simulink model "OFDM_Tx_Rx_Loopback"  (R2020a)
settings: Solver=FixedStepDiscrete  StartTime=0.0  StopTime=inf  RelTol=1e-3
InitFcn:
  | % Set parameters
  | fs = 200e3;
  | 
  | % Load all required variables
  | load('read_addr_data');
  | load('read_addr_cp');
  | load('read_addr_pream');
  | load('read_addr_rx');
  | load('pilot');
  | load('LTSfreq');
  | load('STSfreq');
  | load('LTSread');
  | load('STSread');
  | load('bpsk');
  | load('qpsk');
  | load('qam16');
values from neighbouring files (symbols this model uses):
  bpsk = [0 0 1 1 1 1 0 0 1 0 1 0 ... (48 elements, 48x1)]    [bpsk.mat]
  qam16 = [12 5 10 3 14 8 1 10 8 7 2 13 ... (48 elements, 48x1)]    [qam16.mat]
  qpsk = [1 2 1 2 2 2 3 1 1 3 1 0 ... (48 elements, 48x1)]    [qpsk.mat]
  STSfreq = [0 0 0 0 0 0 0 0 1 0 0 0 ... (64 elements, 1x64)]    [STSfreq.mat]
undefined symbols (not defined in the file or in its folder): data3, LTSfreq, LTSread, pilot, read_addr_cp, read_addr_data, read_addr_pream, read_addr_rx, STSread
libraries: hdlsllib x54, simulink x27, dsphdlxfrm x2, dsphdlsigops x1, dsphdlmathfun x1
(part 1 of 4)
settings Model: Creator=njb13206  LastModifiedBy=njb13206
settings OptimizationCC: BlockReduction=off  ConditionallyExecuteInputs=off  DefaultParameterBehavior=Inlined
settings DebuggingCC: AlgebraicLoopMsg=error  IntegerOverflowMsg=none  ParameterPrecisionLossMsg=none  IntegerSaturationMsg=none
settings HardwareCC: ProdBitPerPointer=32  ProdBitPerSizeT=32  ProdBitPerPtrDiffT=32  ProdLargestAtomicFloat=None  ProdIntDivRoundTo=Undefined  ProdEndianess=Unspecified  ProdWordSize=32  ProdHWDeviceType=ASIC/FPGA->ASIC/FPGA  TargetBitPerPointer=64  TargetBitPerSizeT=64  TargetBitPerPtrDiffT=64  TargetLongLongMode=on  TargetIntDivRoundTo=Zero  TargetEndianess=LittleEndian  TargetWordSize=64  TargetHWDeviceType=Custom Processor->MATLAB Host Computer  ProdEqTarget=off

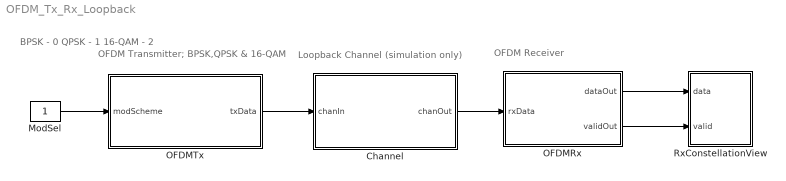
== system OFDM_Tx_Rx_Loopback ==
  note: OFDM Receiver
  note: Loopback Channel (simulation only)
  note: OFDM Transmitter; BPSK,QPSK & 16-QAM
  note: BPSK - 0
      | QPSK - 1
      | 16-QAM - 2
  "Channel " : Subsystem
  ModSel : Constant  OutDataTypeStr=fixdt(0,2,0)  SampleTime=1/fs
  OFDMRx : Subsystem
  OFDMTx : Subsystem
  RxConstellationView : Subsystem
  wires:
  "Channel "/1(chanOut) -> OFDMRx/1(rxData)
  OFDMTx/1(txData) -> "Channel "/1(chanIn)
  OFDMRx/1(dataOut) -> RxConstellationView/1(data)
  OFDMRx/2(validOut) -> RxConstellationView/2(valid)
  ModSel/1 -> OFDMTx/1(modScheme)

== system OFDM_Tx_Rx_Loopback/Channel  ==
  chanIn : Inport
  Delay : Delay  DelayLength=5
  Gain : Gain  Gain=0.1  OutDataTypeStr=fixdt(1,16,14)
  chanOut : Outport  VectorParamsAs1DForOutWhenUnconnected=off
  wires:
  Delay/1 -> chanOut/1
  chanIn/1 -> Gain/1
  Gain/1 -> Delay/1

== system OFDM_Tx_Rx_Loopback/OFDMRx ==
  note: One Tap Equaliser
  note: FFT Demodulation
  note: Timing and Frequency
      | synchronisation
  rxData : Inport
  ChannelEstEq : Subsystem
  FFT : Subsystem
  Synchronisation : Subsystem
  dataOut : Outport  VectorParamsAs1DForOutWhenUnconnected=off
  validOut : Outport  Port=2  VectorParamsAs1DForOutWhenUnconnected=off
  wires:
  rxData/1 -> Synchronisation/1(dataIn)
  FFT/1(dataOut) -> ChannelEstEq/1(dataIn)
  FFT/3(preambleValidOut) -> ChannelEstEq/3(preambleValid)
  FFT/2(dataValidOut) -> ChannelEstEq/2(dataValid)
  Synchronisation/1(DataOut) -> FFT/1(dataIn)
  Synchronisation/2(FFTValidOut) -> FFT/2(FFTValidIn)
  Synchronisation/3(dataValid) -> FFT/3(dataValid)
  Synchronisation/4(preambleValid) -> FFT/4(preambleValid)
  ChannelEstEq/1(dataOut) -> dataOut/1
  ChannelEstEq/2(dataValidOut) -> validOut/1

== system OFDM_Tx_Rx_Loopback/OFDMTx ==
  note: Generate random integers, M-QAM symbol mapping and sub-carrier
      | mapping.
  note: Add Cyclic Prefix
  note: Create OFDM symbols using
      | IFFT
  modScheme : Inport
  CPAdd : Subsystem
  Constant : Constant  OutDataTypeStr=boolean  SampleTime=1/fs
  ControlSignalGenerator : Subsystem
  DataGenerator : Subsystem
  IFFT : Subsystem
  SCMapper : Subsystem
  txData : Outport  VectorParamsAs1DForOutWhenUnconnected=off
  wires:
  DataGenerator/1(dataOut) -> SCMapper/1(dataIn)
  DataGenerator/2(preambValOut) -> SCMapper/2(preambValid)
  DataGenerator/3(dataValidOut) -> SCMapper/3(dataValid)
  SCMapper/1(dataOut) -> IFFT/1(dataIn)
  SCMapper/2(preambValidOut) -> IFFT/2(preambleValidIn)
  SCMapper/3(dataValidOut) -> IFFT/3("dataValidIn ")
  IFFT/1(dataOut) -> CPAdd/1(dataIn)
  IFFT/2(preambValidOut) -> CPAdd/2(preambValid)
  IFFT/3(dataValidOut) -> CPAdd/3(dataValid)
  CPAdd/1(dataOut) -> txData/1
  ControlSignalGenerator/1(dataValid) -> DataGenerator/2(dataValid)
  ControlSignalGenerator/2(preambleValid) -> DataGenerator/3(preambleValid)
  ControlSignalGenerator/3(dataReady) -> DataGenerator/4(dataReady)
  ControlSignalGenerator/4(PilotValid) -> DataGenerator/5(pilotValid)
  modScheme/1 -> DataGenerator/1(modScheme)
  Constant/1 -> ControlSignalGenerator/1(enable)

== system OFDM_Tx_Rx_Loopback/RxConstellationView ==
  data : Inport
  valid : Inport  Port=2
  Constant : Constant  Value=NaN + 1i*NaN  OutDataTypeStr=double  SampleTime=-1
  Constellation Diagram : ConstellationDiagram
  Switch : Switch  Criteria=u2 ~= 0
  wires:
  Switch/1 -> Constellation Diagram/1
  Constant/1 -> Switch/3
  valid/1 -> Switch/2
  data/1 -> Switch/1

== system OFDM_Tx_Rx_Loopback/OFDMRx/ChannelEstEq ==
  dataIn : Inport
  dataValid : Inport  Port=2
  preambleValid : Inport  Port=3
  ChannelEstimate : Subsystem
  DataArrange : Subsystem
  Delay : Delay  DelayLength=6
  Equalise : Subsystem
  dataOut : Outport  VectorParamsAs1DForOutWhenUnconnected=off
  dataValidOut : Outport  Port=2  VectorParamsAs1DForOutWhenUnconnected=off
  wires:
  ChannelEstimate/2(dataValidOut) -> Equalise/3(dataValidIn)
  ChannelEstimate/1(chEstOut) -> Equalise/2(chEstIn)
  Delay/1 -> Equalise/1(dataInEq)
  dataIn/1 -> ChannelEstimate/1(dataIn), Delay/1
  preambleValid/1 -> ChannelEstimate/2(preambleValid)
  dataValid/1 -> ChannelEstimate/3(dataValidIn)
  Equalise/1(dataOutEq) -> DataArrange/1(dataIn)
  Equalise/2(dataValidOut) -> DataArrange/2(validIn)
  DataArrange/1(dataOut) -> dataOut/1
  DataArrange/2(validOut) -> dataValidOut/1

== system OFDM_Tx_Rx_Loopback/OFDMRx/FFT ==
  dataIn : Inport
  FFTValidIn : Inport  Port=2
  dataValid : Inport  Port=3
  preambleValid : Inport  Port=4
  Delay1 : Delay  DelayLength=173
  Delay2 : Delay  DelayLength=173
  FFT HDL Optimized : dsphdlxfrm/FFT HDL Optimized  FFTLength=64  Architecture=Streaming Radix 2^2  ComplexMultiplication=Use 4 multipliers and 2 adders  BitReversedOutput=off  BitReversedInput=off  Normalize=off  SimulateUsing=Code generation  RoundingMethod=Floor  ResetInputPort=off  StartOutputPort=off  EndOutputPort=off
      settings: SourceProductBaseCode=DS
  Terminator : Terminator
  dataOut : Outport  VectorParamsAs1DForOutWhenUnconnected=off
  dataValidOut : Outport  Port=2  VectorParamsAs1DForOutWhenUnconnected=off
  preambleValidOut : Outport  Port=3  VectorParamsAs1DForOutWhenUnconnected=off
  wires:
  FFTValidIn/1 -> FFT HDL Optimized/2
  dataIn/1 -> FFT HDL Optimized/1
  Delay2/1 -> dataValidOut/1
  Delay1/1 -> preambleValidOut/1
  FFT HDL Optimized/1 -> dataOut/1
  FFT HDL Optimized/2 -> Terminator/1
  dataValid/1 -> Delay2/1
  preambleValid/1 -> Delay1/1

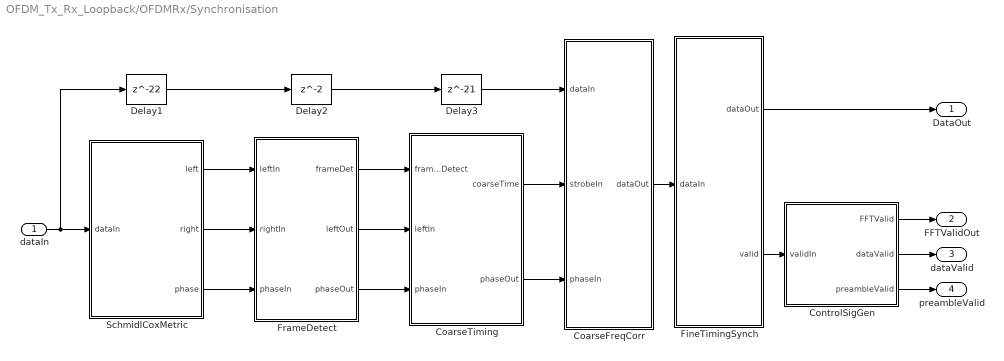
== system OFDM_Tx_Rx_Loopback/OFDMRx/Synchronisation ==
  dataIn : Inport
  CoarseFreqCorr : Subsystem
  CoarseTiming : Subsystem
  ControlSigGen : Subsystem
  Delay1 : Delay  DelayLength=22  InputProcessing=Columns as channels (frame based)
  Delay2 : Delay  InputProcessing=Columns as channels (frame based)
  Delay3 : Delay  DelayLength=21  InputProcessing=Columns as channels (frame based)
  FineTimingSynch : Subsystem
  FrameDetect : Subsystem
  "SchmidlCoxMetric " : Subsystem
  DataOut : Outport  VectorParamsAs1DForOutWhenUnconnected=off
  FFTValidOut : Outport  Port=2  VectorParamsAs1DForOutWhenUnconnected=off
  dataValid : Outport  Port=3  VectorParamsAs1DForOutWhenUnconnected=off
  preambleValid : Outport  Port=4  VectorParamsAs1DForOutWhenUnconnected=off
  wires:
  Delay1/1 -> Delay2/1
  "SchmidlCoxMetric "/3(phase) -> FrameDetect/3(phaseIn)
  "SchmidlCoxMetric "/2(right) -> FrameDetect/2(rightIn)
  FineTimingSynch/1(dataOut) -> DataOut/1
  FrameDetect/2(leftOut) -> CoarseTiming/2(leftIn)
  Delay2/1 -> Delay3/1
  FrameDetect/1(frameDet) -> CoarseTiming/1(frameDetect)
  FrameDetect/3(phaseOut) -> CoarseTiming/3(phaseIn)
  CoarseTiming/1(coarseTime) -> CoarseFreqCorr/2(strobeIn)
  dataIn/1 -> "SchmidlCoxMetric "/1(dataIn), Delay1/1
  Delay3/1 -> CoarseFreqCorr/1(dataIn)
  "SchmidlCoxMetric "/1(left) -> FrameDetect/1(leftIn)
  CoarseFreqCorr/1(dataOut) -> FineTimingSynch/1(dataIn)
  CoarseTiming/2(phaseOut) -> CoarseFreqCorr/3(phaseIn)
  ControlSigGen/1(FFTValid) -> FFTValidOut/1
  FineTimingSynch/2(valid) -> ControlSigGen/1(validIn)
  ControlSigGen/2(dataValid) -> dataValid/1
  ControlSigGen/3(preambleValid) -> preambleValid/1

== system OFDM_Tx_Rx_Loopback/OFDMTx/CPAdd ==
  dataIn : Inport
  preambValid : Inport  Port=2
  dataValid : Inport  Port=3
  DataExtend : Subsystem
  LTFExtend : Subsystem
  Mux2 : MATLAB Function  TreatAsAtomicUnit=on
  STFExtend : Subsystem
  dataOut : Outport  VectorParamsAs1DForOutWhenUnconnected=off
  wires:
  preambValid/1 -> LTFExtend/2(preambVal), STFExtend/2(preambVal)
  dataIn/1 -> DataExtend/1(dataIn), LTFExtend/1(data), STFExtend/1(data)
  STFExtend/1(STFExtendOut) -> Mux2/1(sts)
  STFExtend/2(STFValidOut) -> Mux2/2(stsval)
  LTFExtend/1(LTFExtendOut) -> Mux2/3(lts)
  LTFExtend/2(LTFValidOut) -> Mux2/4(ltsval)
  DataExtend/1(dataOut) -> Mux2/5(data)
  DataExtend/2(dataValidOut) -> Mux2/6(dataval)
  Mux2/1(dataOut) -> dataOut/1
  dataValid/1 -> DataExtend/2(dataValid)

== system OFDM_Tx_Rx_Loopback/OFDMTx/ControlSignalGenerator ==
  enable : Inport
  PreamValidGen : Subsystem
  dataReadyGen : Subsystem
  dataValidGen : Subsystem
  pilotValidGen : Subsystem
  dataValid : Outport
  preambleValid : Outport  Port=2
  dataReady : Outport  Port=3
  PilotValid : Outport  Port=4
  wires:
  enable/1 -> dataValidGen/2(enable), PreamValidGen/1(enable)
  dataReadyGen/1(y) -> dataReady/1
  pilotValidGen/1(y) -> PilotValid/1
  PreamValidGen/1(y) -> preambleValid/1, dataValidGen/1(y)
  dataValidGen/1(valOut) -> pilotValidGen/1(enb), dataReadyGen/1(enb), dataValid/1

== system OFDM_Tx_Rx_Loopback/OFDMTx/DataGenerator ==
  modScheme : Inport
  dataValid : Inport  Port=2
  preambleValid : Inport  Port=3
  dataReady : Inport  Port=4
  pilotValid : Inport  Port=5
  Data Multiplexer : MATLAB Function  TreatAsAtomicUnit=on
  LTSfreq : Subsystem
  PilotGen : Subsystem
  STSFreq : Subsystem
  SymbolsGen : Subsystem
  dataOut : Outport  VectorParamsAs1DForOutWhenUnconnected=off
  preambValOut : Outport  Port=2  VectorParamsAs1DForOutWhenUnconnected=off
  dataValidOut : Outport  Port=3  VectorParamsAs1DForOutWhenUnconnected=off
  wires:
  SymbolsGen/1(symbsOut) -> Data Multiplexer/1(symbols)
  LTSfreq/1(ltsFreq) -> Data Multiplexer/7(lts)
  LTSfreq/2(ltsVal) -> Data Multiplexer/8(ltsval)
  PilotGen/1(pilotOut) -> Data Multiplexer/3(pilots)
  STSFreq/1(stsFreq) -> Data Multiplexer/5(sts)
  STSFreq/2(stsVal) -> Data Multiplexer/6(stsval)
  Data Multiplexer/1(data) -> dataOut/1
  dataValid/1 -> dataValidOut/1, PilotGen/1(dataValidIn)
  preambleValid/1 -> STSFreq/1(preamVal), LTSfreq/1(preambVal), preambValOut/1
  dataReady/1 -> SymbolsGen/2(valid), Data Multiplexer/2(dataready)
  pilotValid/1 -> PilotGen/2(pilotValidIn), Data Multiplexer/4(pval)
  modScheme/1 -> SymbolsGen/1(modScheme)

== system OFDM_Tx_Rx_Loopback/OFDMTx/IFFT ==
  dataIn : Inport
  preambleValidIn : Inport  Port=2
  "dataValidIn " : Inport  Port=3
  Delay : Delay  DelayLength=173  InitialCondition=0  UseCircularBuffer=on
  Delay1 : Delay  DelayLength=173  InitialCondition=0  UseCircularBuffer=on
  IFFT HDL Optimized : dsphdlxfrm/IFFT HDL Optimized  FFTLength=64  Architecture=Streaming Radix 2^2  ComplexMultiplication=Use 3 multipliers and 5 adders  BitReversedOutput=off  BitReversedInput=off  Normalize=on  SimulateUsing=Code generation  RoundingMethod=Floor  ResetInputPort=off  StartOutputPort=off  EndOutputPort=off
      settings: SourceProductBaseCode=DS
  IFFTValid : Subsystem
  Terminator : Terminator
  dataOut : Outport  VectorParamsAs1DForOutWhenUnconnected=off
  preambValidOut : Outport  Port=2  VectorParamsAs1DForOutWhenUnconnected=off
  dataValidOut : Outport  Port=3  VectorParamsAs1DForOutWhenUnconnected=off
  wires:
  dataIn/1 -> IFFT HDL Optimized/1
  IFFT HDL Optimized/2 -> Terminator/1
  "dataValidIn "/1 -> IFFTValid/2(dataValid), Delay1/1
  IFFTValid/1(ifftValid) -> IFFT HDL Optimized/2
  preambleValidIn/1 -> IFFTValid/1(preambleValid), Delay/1
  Delay/1 -> preambValidOut/1
  Delay1/1 -> dataValidOut/1
  IFFT HDL Optimized/1 -> dataOut/1

== system OFDM_Tx_Rx_Loopback/OFDMTx/SCMapper ==
  dataIn : Inport
  preambValid : Inport  Port=2
  dataValid : Inport  Port=3
  DataMapper : Subsystem
  Mux2 : MATLAB Function  TreatAsAtomicUnit=on
  PremableMapper : Subsystem
  dataOut : Outport  VectorParamsAs1DForOutWhenUnconnected=off
  preambValidOut : Outport  Port=2  VectorParamsAs1DForOutWhenUnconnected=off
  dataValidOut : Outport  Port=3  VectorParamsAs1DForOutWhenUnconnected=off
  wires:
  PremableMapper/1(preambleShiftOut) -> Mux2/1(preamb)
  PremableMapper/2(preambValOut) -> preambValidOut/1, Mux2/2(preambVal)
  DataMapper/1(dataOut) -> Mux2/3(data)
  DataMapper/2(dataValidOut) -> dataValidOut/1, Mux2/4(dataVal)
  dataIn/1 -> DataMapper/1(dataIn), PremableMapper/1(data)
  preambValid/1 -> PremableMapper/2(preambVal)
  dataValid/1 -> DataMapper/2(dataValid)
  Mux2/1(dataOut) -> dataOut/1

== system OFDM_Tx_Rx_Loopback/OFDMRx/ChannelEstEq/ChannelEstimate ==
  note: Note the preamble symbols do not pass this point.
  note: Write averaged channel estimate to RAM and read out when data is valid
      | for equalisation of successive OFDM symbols.
  note: Get and store the channel estimate using the two
      | repetitions of the L-LTF
  dataIn : Inport
  preambleValid : Inport  Port=2
  dataValidIn : Inport  Port=3
  ChanEst : Subsystem
  Delay : Delay  DelayLength=5
  Delay1 : Delay  DelayLength=5
  Delay2 : Delay  DelayLength=1
  Dual Port RAM1 : hdlsllib/HDL RAMs/Dual Port RAM  ram_size=6
      settings: SourceProductBaseCode=SL
  HDL Counter3 : hdlsllib/Sources/HDL Counter  CountType=Count limited  CountInit=0  CountStep=1  CountMax=63  CountFromType=Initial value  CountFrom=0  CountResetPort=off  CountLoadPort=off  CountEnbPort=on  CountDirPort=off  CountDataType=Unsigned  CountWordLen=6  CountFracLen=0  CountSampTime=1
  Terminator : Terminator
  WriteEnbAddrGen : Subsystem
  chEstOut : Outport  VectorParamsAs1DForOutWhenUnconnected=off
  dataValidOut : Outport  Port=2  VectorParamsAs1DForOutWhenUnconnected=off
  wires:
  HDL Counter3/1 -> Dual Port RAM1/4
  Dual Port RAM1/2 -> chEstOut/1
  Delay2/1 -> dataValidOut/1
  preambleValid/1 -> ChanEst/2(PreambValidIn), Delay/1
  dataIn/1 -> ChanEst/1(ChanEstIn)
  ChanEst/1(ChEstOut) -> Dual Port RAM1/1
  dataValidIn/1 -> Delay1/1
  Delay1/1 -> HDL Counter3/1, Delay2/1
  Delay/1 -> WriteEnbAddrGen/1(In1)
  WriteEnbAddrGen/1(Out1) -> Dual Port RAM1/2
  WriteEnbAddrGen/2(Out2) -> Dual Port RAM1/3
  Dual Port RAM1/1 -> Terminator/1

== system OFDM_Tx_Rx_Loopback/OFDMRx/ChannelEstEq/DataArrange ==
  dataIn : Inport
  validIn : Inport  Port=2
  Compare To Constant4 : simulink/Logic and Bit Operations/Compare To Constant  relop=>=  const=17  OutDataTypeStr=boolean
  Compare To Constant5 : simulink/Logic and Bit Operations/Compare To Constant  relop=<=  const=64  OutDataTypeStr=boolean
  Data Type Conversion : DataTypeConversion  OutDataTypeStr=fixdt(1,16,14)
  Logical Operator2 : Logic  IconShape=distinctive  AllPortsSameDT=off  OutDataTypeStr=boolean
  SCReArrange : Subsystem
  SampleCounter : Subsystem
  dataOut : Outport
  validOut : Outport  Port=2
  wires:
  SampleCounter/1(Sample_Cnt) -> Compare To Constant4/1, Compare To Constant5/1
  Compare To Constant4/1 -> Logical Operator2/1
  Compare To Constant5/1 -> Logical Operator2/2
  SCReArrange/2(DataValidOut) -> SampleCounter/1(Valid_In)
  dataIn/1 -> SCReArrange/1(DataIn)
  validIn/1 -> SCReArrange/2(DataValidIn)
  SCReArrange/1(DataOut) -> Data Type Conversion/1
  Logical Operator2/1 -> validOut/1
  Data Type Conversion/1 -> dataOut/1

== system OFDM_Tx_Rx_Loopback/OFDMRx/ChannelEstEq/Equalise ==
  dataInEq : Inport
  chEstIn : Inport  Port=2
  dataValidIn : Inport  Port=3
  Abs2 : Subsystem
  Complex Mult : Subsystem
  Delay1 : Delay
  Delay8 : Delay  DelayLength=3
  Divide : Subsystem
  dataOutEq : Outport  VectorParamsAs1DForOutWhenUnconnected=off
  dataValidOut : Outport  Port=2  VectorParamsAs1DForOutWhenUnconnected=off
  wires:
  dataValidIn/1 -> Delay8/1
  chEstIn/1 -> Abs2/1(ChEstIn), Complex Mult/2(In2)
  dataInEq/1 -> Complex Mult/1(In1)
  Complex Mult/1(Out1) -> Divide/1(In1)
  Abs2/1(Out1) -> Divide/2(In2)
  Divide/1(Out1) -> dataOutEq/1
  Delay8/1 -> Delay1/1
  Delay1/1 -> dataValidOut/1

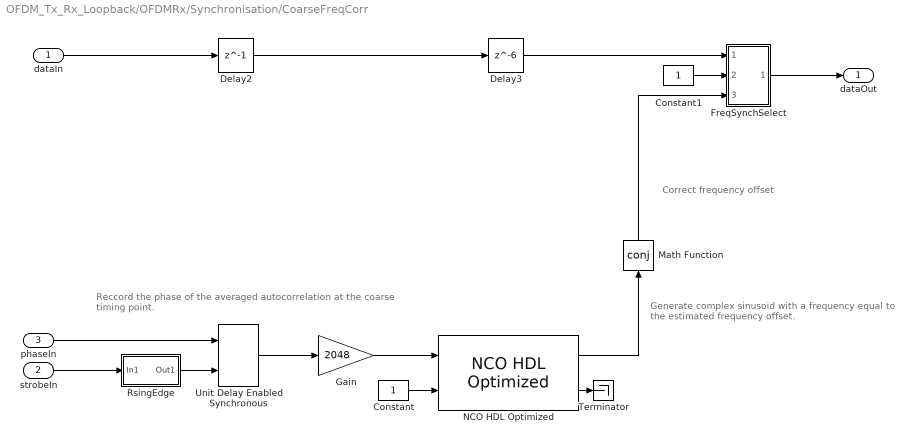
== system OFDM_Tx_Rx_Loopback/OFDMRx/Synchronisation/CoarseFreqCorr ==
  note: Generate complex sinusoid with a frequency equal
      | to the estimated frequency offset.
  note: Correct frequency offset
  note: Reccord the phase of the averaged autocorrelation at the coarse
      | timing point.
  dataIn : Inport
  strobeIn : Inport  Port=2
  phaseIn : Inport  Port=3
  Constant : Constant  VectorParams1D=off  OutDataTypeStr=boolean  SampleTime=1/fs
  Constant1 : Constant  OutDataTypeStr=fixdt(0,1,0)  SampleTime=1/fs
  Delay2 : Delay  DelayLength=1
  Delay3 : Delay  DelayLength=6
  FreqSynchSelect : Subsystem
  Gain : Gain  Gain=2048  OutDataTypeStr=uint16
  Math Function : Math  Operator=conj  SignedPower=on  RndMeth=Zero  SaturateOnIntegerOverflow=on
  NCO HDL Optimized : dsphdlsigops/NCO HDL Optimized  PhaseIncrementSource=Input port  PhaseIncrement=100  PhaseOffsetSource=Property  PhaseOffset=0  DitherSource=Property  NumDitherBits=4  SamplesPerFrame=1  LUTCompress=on  ResetAction=off  Waveform=Complex exponential  PhasePort=off  SimulateUsing=Code generation  AccumulatorWL=16  PhaseQuantization=on  NumQuantizerAccumulatorBits=12  OutputDataType=Binary point scaling  OutputWL=16  OutputFL=14
      settings: SourceProductBaseCode=DS
  RsingEdge : Subsystem
  Terminator : Terminator
  Unit Delay Enabled Synchronous : hdlsllib/Discrete/Unit Delay Enabled Synchronous  InitialCondition=0.0  SampleTime=-1
      settings: SourceProductBaseCode=SL
  dataOut : Outport  VectorParamsAs1DForOutWhenUnconnected=off
  wires:
  Constant/1 -> NCO HDL Optimized/2
  NCO HDL Optimized/2 -> Terminator/1
  NCO HDL Optimized/1 -> Math Function/1
  Gain/1 -> NCO HDL Optimized/1
  Unit Delay Enabled Synchronous/1 -> Gain/1
  Delay2/1 -> Delay3/1
  strobeIn/1 -> RsingEdge/1(In1)
  RsingEdge/1(Out1) -> Unit Delay Enabled Synchronous/2
  phaseIn/1 -> Unit Delay Enabled Synchronous/1
  dataIn/1 -> Delay2/1
  Delay3/1 -> FreqSynchSelect/1(In1)
  Math Function/1 -> FreqSynchSelect/3(In3)
  FreqSynchSelect/1(Out1) -> dataOut/1
  Constant1/1 -> FreqSynchSelect/2(In2)

== system OFDM_Tx_Rx_Loopback/OFDMRx/Synchronisation/CoarseTiming ==
  note: When the frame is detected, the frame detected strobe goes high and remains in this state
      | until a reset is supplied. The coarse timing is determined by seraching for the maximum value
      | of |P(d)|^2 in a window of 20 samples after the packet starting point. The index of this sample
      | corresponds to the coarse timing point.
      |
      | Due to the plateau effect associated with the S&C metric, the coarse timing is not used for
      | sample level synchronisation. However, the phase of the averaged autocorrelation at the
      | coarse timing point can be used as a coarse estimate of the CFO.
      |
      | Sample level synchronisation is achieved using a matched filter with coefficients corresponding
      | to the time-reversed and conjugated L-LTF.
  frameDetect : Inport
  leftIn : Inport  Port=2
  phaseIn : Inport  Port=3
  CoarseTimeStrobeGen : Subsystem
  Delay : Delay  DelayLength=21  InitialCondition=0  UseCircularBuffer=on
  coarseTime : Outport  VectorParamsAs1DForOutWhenUnconnected=off
  phaseOut : Outport  Port=2  VectorParamsAs1DForOutWhenUnconnected=off
  wires:
  Delay/1 -> phaseOut/1
  CoarseTimeStrobeGen/1(coarseStrobeOut) -> coarseTime/1
  phaseIn/1 -> Delay/1
  frameDetect/1 -> CoarseTimeStrobeGen/2(packetDet)
  leftIn/1 -> CoarseTimeStrobeGen/1(dataIn)

== system OFDM_Tx_Rx_Loopback/OFDMRx/Synchronisation/ControlSigGen ==
  validIn : Inport
  OR : Logic  Operator=OR  IconShape=distinctive  AllPortsSameDT=off  OutDataTypeStr=boolean
  PreambleValidGen : Subsystem
  dataValidGen : Subsystem
  FFTValid : Outport  VectorParamsAs1DForOutWhenUnconnected=off
  dataValid : Outport  Port=2  VectorParamsAs1DForOutWhenUnconnected=off
  preambleValid : Outport  Port=3  VectorParamsAs1DForOutWhenUnconnected=off
  wires:
  validIn/1 -> dataValidGen/2(enb1), PreambleValidGen/1(ValidIn)
  PreambleValidGen/1(y) -> preambleValid/1, OR/1, dataValidGen/1(enb)
  dataValidGen/1(y) -> OR/2, dataValid/1
  OR/1 -> FFTValid/1

== system OFDM_Tx_Rx_Loopback/OFDMRx/Synchronisation/FineTimingSynch ==
  note: The threshold for the matched filter is the signal energy which is measured
      | over a block of 64 samples.
  note: This entity is responsible for fine timing synchronisation. This is achieved using a matched filter
      | with coefficients that are a time-reversed and conjugated version of the L-LTF. In this implementation,
      |  the quantised L-LTF is used in order to reduce the cost of the correlation in terms of embedded
      | multipliers.
  note: The abs^2 of the correlation is compared to a threshold in order
      | to achieve sample level synchronisation. The first sample to
      | exceed the threshold should correspond to the middle of the two
      | repetitions of the L-LTF. When this occurs, the data valid signal is
      | generated and this is used to start the FFT demodulation process.
  dataIn : Inport
  Abs1 : Subsystem
  Abs2 : Subsystem
  Delay1 : Delay  DelayLength=1
  Delay2 : Delay  DelayLength=64
  Delay3 : Delay  DelayLength=64
  Delay4 : Delay
  MatchedFilter : Subsystem
      mask help: Matched filter with coeffients equal to quantised version of time reversed and conjugated L-LTF.
  MovingAvg : Subsystem
  threshCompare : Subsystem
  dataOut : Outport
  valid : Outport  Port=2
  wires:
  Delay4/1 -> Delay1/1
  Delay1/1 -> Delay2/1
  threshCompare/1(Out1) -> valid/1
  Delay2/1 -> dataOut/1
  Delay3/1 -> Delay4/1
  Abs2/1(Out1) -> threshCompare/1(In1)
  Abs1/1(Out1) -> MovingAvg/1(DataIn)
  MovingAvg/1(Out1) -> threshCompare/2(In2)
  MatchedFilter/1(dataOut) -> Abs2/1(dataOut)
  dataIn/1 -> Abs1/1(DataIn), MatchedFilter/1(dataIn), Delay3/1

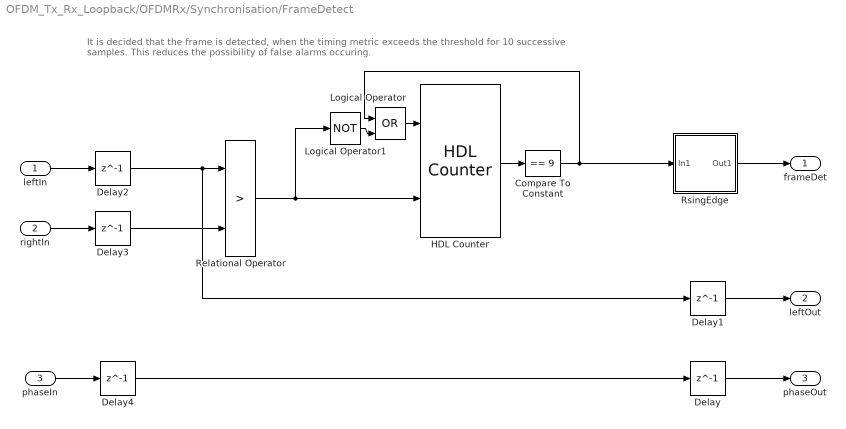
== system OFDM_Tx_Rx_Loopback/OFDMRx/Synchronisation/FrameDetect ==
  note: It is decided that the frame is detected, when the timing metric exceeds the threshold for 10 successive samples.
      | This reduces the possibility of false alarms occuring.
  leftIn : Inport
  rightIn : Inport  Port=2
  phaseIn : Inport  Port=3
  Compare To Constant : simulink/Logic and Bit Operations/Compare To Constant  relop===  const=9  OutDataTypeStr=boolean
  Delay{,1..4} (5 alike) : Delay  DelayLength=1
  HDL Counter : hdlsllib/Sources/HDL Counter  CountType=Count limited  CountInit=0  CountStep=1  CountMax=9  CountFromType=Initial value  CountFrom=0  CountResetPort=on  CountLoadPort=off  CountEnbPort=on  CountDirPort=off  CountDataType=Unsigned  CountWordLen=4  CountFracLen=0  CountSampTime=1
  Logical Operator : Logic  Operator=OR  IconShape=distinctive  AllPortsSameDT=off  OutDataTypeStr=boolean
  Logical Operator1 : Logic  Operator=NOT  IconShape=distinctive  AllPortsSameDT=off  OutDataTypeStr=boolean
  Relational Operator : RelationalOperator  Operator=>  OutDataTypeStr=boolean  RndMeth=Simplest
  RsingEdge : Subsystem
  frameDet : Outport  VectorParamsAs1DForOutWhenUnconnected=off
  leftOut : Outport  Port=2  VectorParamsAs1DForOutWhenUnconnected=off
  phaseOut : Outport  Port=3  VectorParamsAs1DForOutWhenUnconnected=off
  wires:
  Delay4/1 -> Delay/1
  Delay2/1 -> Relational Operator/1, Delay1/1
  RsingEdge/1(Out1) -> frameDet/1
  Delay/1 -> phaseOut/1
  Delay1/1 -> leftOut/1
  leftIn/1 -> Delay2/1
  phaseIn/1 -> Delay4/1
  Logical Operator/1 -> HDL Counter/1
  Compare To Constant/1 -> Logical Operator/1, RsingEdge/1(In1)
  HDL Counter/1 -> Compare To Constant/1
  rightIn/1 -> Delay3/1
  Logical Operator1/1 -> Logical Operator/2
  Relational Operator/1 -> Logical Operator1/1, HDL Counter/2
  Delay3/1 -> Relational Operator/2

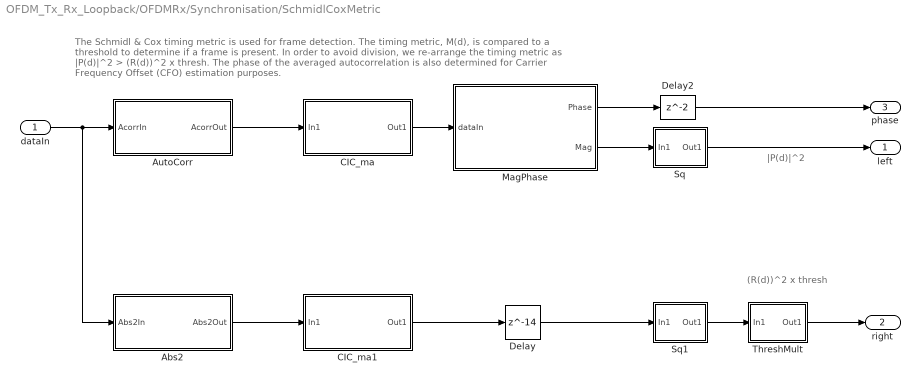
== system OFDM_Tx_Rx_Loopback/OFDMRx/Synchronisation/SchmidlCoxMetric  ==
  note: (R(d))^2 x thresh
  note: |P(d)|^2
  note: The Schmidl & Cox timing metric is used for frame detection. The timing metric, M(d), is compared to a threshold
      | to determine if a frame is present. In order to avoid division, we re-arrange the timing metric as |P(d)|^2 > (R(d))^2 x thresh.
      | The phase of the averaged autocorrelation is also determined for Carrier Frequency Offset (CFO) estimation purposes.
  dataIn : Inport
  Abs2 : Subsystem
  AutoCorr : Subsystem
  CIC_ma : Subsystem
  CIC_ma1 : Subsystem
  Delay : Delay  DelayLength=14
  Delay2 : Delay
  MagPhase : Subsystem
  Sq : Subsystem
  Sq1 : Subsystem
  ThreshMult : Subsystem
  left : Outport  VectorParamsAs1DForOutWhenUnconnected=off
  right : Outport  Port=2  VectorParamsAs1DForOutWhenUnconnected=off
  phase : Outport  Port=3  VectorParamsAs1DForOutWhenUnconnected=off
  wires:
  MagPhase/1(Phase) -> Delay2/1
  Delay2/1 -> phase/1
  CIC_ma/1(Out1) -> MagPhase/1(dataIn)
  AutoCorr/1(AcorrOut) -> CIC_ma/1(In1)
  MagPhase/2(Mag) -> Sq/1(In1)
  Abs2/1(Abs2Out) -> CIC_ma1/1(In1)
  dataIn/1 -> Abs2/1(Abs2In), AutoCorr/1(AcorrIn)
  CIC_ma1/1(Out1) -> Delay/1
  Delay/1 -> Sq1/1(In1)
  Sq1/1(Out1) -> ThreshMult/1(In1)
  ThreshMult/1(Out1) -> right/1
  Sq/1(Out1) -> left/1

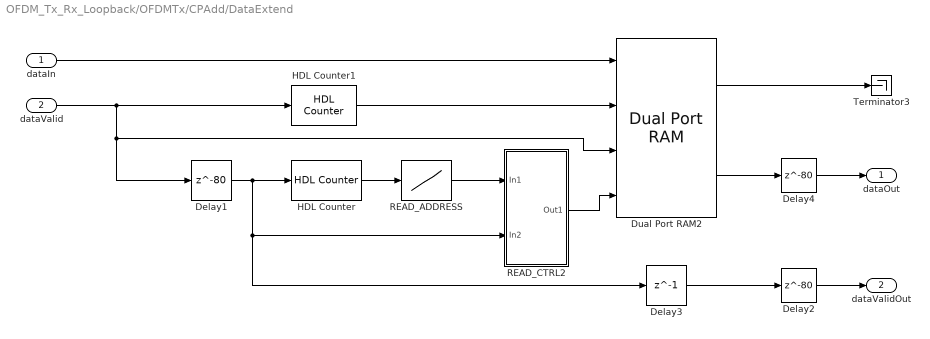
== system OFDM_Tx_Rx_Loopback/OFDMTx/CPAdd/DataExtend ==
  dataIn : Inport
  dataValid : Inport  Port=2
  Delay1 : Delay  DelayLength=80  InitialCondition=0  UseCircularBuffer=on
  Delay2 : Delay  DelayLength=80
  Delay3 : Delay  DelayLength=1  InitialCondition=0  UseCircularBuffer=on
  Delay4 : Delay  DelayLength=80
  Dual Port RAM2 : hdlsllib/HDL RAMs/Dual Port RAM  ram_size=8
      settings: SourceProductBaseCode=SL
  HDL Counter : hdlsllib/Sources/HDL Counter  CountType=Count limited  CountInit=0  CountStep=1  CountMax=159  CountFromType=Initial value  CountFrom=0  CountResetPort=off  CountLoadPort=off  CountEnbPort=on  CountDirPort=off  CountDataType=Unsigned  CountWordLen=8  CountFracLen=0  CountSampTime=1
  HDL Counter1 : hdlsllib/Sources/HDL Counter  CountType=Count limited  CountInit=0  CountStep=1  CountMax=159  CountFromType=Initial value  CountFrom=0  CountResetPort=off  CountLoadPort=off  CountEnbPort=on  CountDirPort=off  CountDataType=Unsigned  CountWordLen=8  CountFracLen=0  CountSampTime=1
  READ_ADDRESS : Lookup_n-D  NumberOfTableDimensions=1  LookupTableObject=''  BreakpointsForDimension1=[0:159]  BreakpointsForDimension1FirstPoint=10  BreakpointsForDimension2FirstPoint=10  BreakpointsForDimension1Spacing=12  BreakpointsForDimension2Spacing=12  IndexSearchMethod=Evenly spaced points  Table=read_addr_cp  TableDataTypeStr=fixdt(0,8,0)  InterpMethod=Flat  DiagnosticForOutOfRangeInput=Error  InternalRulePriority=Speed  OutDataTypeStr=fixdt(0,8,0)  RndMeth=Simplest  InputSameDT=on
  READ_CTRL2 : Subsystem
  Terminator3 : Terminator
  dataOut : Outport  VectorParamsAs1DForOutWhenUnconnected=off
  dataValidOut : Outport  Port=2  VectorParamsAs1DForOutWhenUnconnected=off
  wires:
  Delay4/1 -> dataOut/1
  Delay2/1 -> dataValidOut/1
  Dual Port RAM2/1 -> Terminator3/1
  READ_ADDRESS/1 -> READ_CTRL2/1(In1)
  HDL Counter/1 -> READ_ADDRESS/1
  dataIn/1 -> Dual Port RAM2/1
  HDL Counter1/1 -> Dual Port RAM2/2
  Delay1/1 -> HDL Counter/1, Delay3/1, READ_CTRL2/2(In2)
  Dual Port RAM2/2 -> Delay4/1
  dataValid/1 -> HDL Counter1/1, Dual Port RAM2/3, Delay1/1
  Delay3/1 -> Delay2/1
  READ_CTRL2/1(Out1) -> Dual Port RAM2/4

== system OFDM_Tx_Rx_Loopback/OFDMTx/CPAdd/LTFExtend ==
  data : Inport
  preambVal : Inport  Port=2
  Delay : Delay  DelayLength=160  InitialCondition=0  UseCircularBuffer=on
  Delay12 : Delay  DelayLength=1  InitialCondition=0  UseCircularBuffer=on
  Dual Port RAM : hdlsllib/HDL RAMs/Dual Port RAM  ram_size=8
      settings: SourceProductBaseCode=SL
  HDL Counter2 : hdlsllib/Sources/HDL Counter  CountType=Count limited  CountInit=0  CountStep=1  CountMax=159  CountFromType=Initial value  CountFrom=0  CountResetPort=off  CountLoadPort=off  CountEnbPort=on  CountDirPort=off  CountDataType=Unsigned  CountWordLen=8  CountFracLen=0  CountSampTime=1
  HDL Counter3 : hdlsllib/Sources/HDL Counter  CountType=Count limited  CountInit=0  CountStep=1  CountMax=159  CountFromType=Initial value  CountFrom=0  CountResetPort=off  CountLoadPort=off  CountEnbPort=on  CountDirPort=off  CountDataType=Unsigned  CountWordLen=8  CountFracLen=0  CountSampTime=1
  LTFValidGen : Subsystem
  READ_CTRL : Subsystem
  Terminator1 : Terminator
  readaddr : Lookup_n-D  NumberOfTableDimensions=1  LookupTableObject=''  BreakpointsForDimension1=0:159  BreakpointsForDimension1FirstPoint=10  BreakpointsForDimension2FirstPoint=10  BreakpointsForDimension1Spacing=12  BreakpointsForDimension2Spacing=12  IndexSearchMethod=Evenly spaced points  Table=LTSread  TableDataTypeStr=fixdt(0,8,0)  InterpMethod=Flat  DiagnosticForOutOfRangeInput=Error  InternalRulePriority=Speed  OutDataTypeStr=fixdt(0,8,0)  RndMeth=Simplest  InputSameDT=on
  LTFExtendOut : Outport  VectorParamsAs1DForOutWhenUnconnected=off
  LTFValidOut : Outport  Port=2  VectorParamsAs1DForOutWhenUnconnected=off
  wires:
  readaddr/1 -> READ_CTRL/1(In1)
  READ_CTRL/1(Out1) -> Dual Port RAM/4
  HDL Counter3/1 -> Dual Port RAM/2
  Delay/1 -> READ_CTRL/2(In2), Delay12/1, HDL Counter2/1
  Dual Port RAM/1 -> Terminator1/1
  Delay12/1 -> LTFValidOut/1
  HDL Counter2/1 -> readaddr/1
  data/1 -> Dual Port RAM/1
  Dual Port RAM/2 -> LTFExtendOut/1
  preambVal/1 -> LTFValidGen/1(In1)
  LTFValidGen/1(Out1) -> Dual Port RAM/3, Delay/1, HDL Counter3/1

== system OFDM_Tx_Rx_Loopback/OFDMTx/CPAdd/STFExtend ==
  data : Inport
  preambVal : Inport  Port=2
  Delay : Delay  DelayLength=160  InitialCondition=0  UseCircularBuffer=on
  Delay12 : Delay  DelayLength=1  InitialCondition=0  UseCircularBuffer=on
  Dual Port RAM : hdlsllib/HDL RAMs/Dual Port RAM  ram_size=8
      settings: SourceProductBaseCode=SL
  HDL Counter2 : hdlsllib/Sources/HDL Counter  CountType=Count limited  CountInit=0  CountStep=1  CountMax=159  CountFromType=Initial value  CountFrom=0  CountResetPort=off  CountLoadPort=off  CountEnbPort=on  CountDirPort=off  CountDataType=Unsigned  CountWordLen=8  CountFracLen=0  CountSampTime=1
  HDL Counter3 : hdlsllib/Sources/HDL Counter  CountType=Count limited  CountInit=0  CountStep=1  CountMax=159  CountFromType=Initial value  CountFrom=0  CountResetPort=off  CountLoadPort=off  CountEnbPort=on  CountDirPort=off  CountDataType=Unsigned  CountWordLen=8  CountFracLen=0  CountSampTime=1
  READ_CTRL : Subsystem
  STFValidGen : Subsystem
  Terminator1 : Terminator
  readaddr : Lookup_n-D  NumberOfTableDimensions=1  LookupTableObject=''  BreakpointsForDimension1=0:159  BreakpointsForDimension1FirstPoint=10  BreakpointsForDimension2FirstPoint=10  BreakpointsForDimension1Spacing=12  BreakpointsForDimension2Spacing=12  IndexSearchMethod=Evenly spaced points  Table=STSread  TableDataTypeStr=fixdt(0,8,0)  InterpMethod=Flat  DiagnosticForOutOfRangeInput=Error  InternalRulePriority=Speed  OutDataTypeStr=fixdt(0,8,0)  RndMeth=Simplest  InputSameDT=on
  STFExtendOut : Outport  VectorParamsAs1DForOutWhenUnconnected=off
  STFValidOut : Outport  Port=2  VectorParamsAs1DForOutWhenUnconnected=off
  wires:
  Dual Port RAM/2 -> STFExtendOut/1
  data/1 -> Dual Port RAM/1
  HDL Counter2/1 -> readaddr/1
  Delay12/1 -> STFValidOut/1
  Dual Port RAM/1 -> Terminator1/1
  Delay/1 -> HDL Counter2/1, Delay12/1, READ_CTRL/2(In2)
  HDL Counter3/1 -> Dual Port RAM/2
  READ_CTRL/1(Out1) -> Dual Port RAM/4
  preambVal/1 -> STFValidGen/1(In1)
  readaddr/1 -> READ_CTRL/1(In1)
  STFValidGen/1(Out1) -> HDL Counter3/1, Dual Port RAM/3, Delay/1

== system OFDM_Tx_Rx_Loopback/OFDMTx/ControlSignalGenerator/PreamValidGen ==
  enable : Inport
  Compare To Constant : simulink/Logic and Bit Operations/Compare To Constant  relop===  const=320  OutDataTypeStr=boolean
  HDL Counter : hdlsllib/Sources/HDL Counter  CountType=Count limited  CountInit=0  CountStep=1  CountMax=320  CountFromType=Initial value  CountFrom=0  CountResetPort=on  CountLoadPort=off  CountEnbPort=on  CountDirPort=off  CountDataType=Unsigned  CountWordLen=9  CountFracLen=0  CountSampTime=1
  NOT : Logic  Operator=NOT  IconShape=distinctive  AllPortsSameDT=off  OutDataTypeStr=boolean
  RisingEdge : Subsystem
  Unit Delay Enabled Resettable Synchronous : hdlsllib/Discrete/Unit Delay Enabled Resettable Synchronous  InitialCondition=0.0  SampleTime=-1
      settings: SourceProductBaseCode=SL
  y : Outport  VectorParamsAs1DForOutWhenUnconnected=off
  wires:
  HDL Counter/1 -> Compare To Constant/1
  RisingEdge/1(Out1) -> Unit Delay Enabled Resettable Synchronous/2
  Compare To Constant/1 -> Unit Delay Enabled Resettable Synchronous/3
  enable/1 -> RisingEdge/1(In1), Unit Delay Enabled Resettable Synchronous/1, NOT/1, HDL Counter/2
  Unit Delay Enabled Resettable Synchronous/1 -> y/1
  NOT/1 -> HDL Counter/1

== system OFDM_Tx_Rx_Loopback/OFDMTx/ControlSignalGenerator/dataReadyGen ==
  enb : Inport
  Compare To Constant : simulink/Logic and Bit Operations/Compare To Constant  relop=>  const=31  OutDataTypeStr=boolean
  HDL Counter : hdlsllib/Sources/HDL Counter  CountType=Count limited  CountInit=0  CountStep=1  CountMax=79  CountFromType=Initial value  CountFrom=0  CountResetPort=on  CountLoadPort=off  CountEnbPort=on  CountDirPort=off  CountDataType=Unsigned  CountWordLen=7  CountFracLen=0  CountSampTime=1
  NOT : Logic  Operator=NOT  IconShape=distinctive  AllPortsSameDT=off  OutDataTypeStr=boolean
  y : Outport
  wires:
  HDL Counter/1 -> Compare To Constant/1
  enb/1 -> NOT/1, HDL Counter/2
  NOT/1 -> HDL Counter/1
  Compare To Constant/1 -> y/1

== system OFDM_Tx_Rx_Loopback/OFDMTx/ControlSignalGenerator/dataValidGen ==
  y : Inport
  enable : Inport  Port=2
  AND : Logic  IconShape=distinctive  AllPortsSameDT=off  OutDataTypeStr=boolean
  Delay : Delay  DelayLength=1
  NOT : Logic  Operator=NOT  IconShape=distinctive  AllPortsSameDT=off  OutDataTypeStr=boolean
  valOut : Outport
  wires:
  NOT/1 -> AND/1
  Delay/1 -> AND/2
  AND/1 -> valOut/1
  y/1 -> NOT/1
  enable/1 -> Delay/1

== system OFDM_Tx_Rx_Loopback/OFDMTx/ControlSignalGenerator/pilotValidGen ==
  enb : Inport
  AND : Logic  IconShape=distinctive  AllPortsSameDT=off  OutDataTypeStr=boolean
  Compare To Constant : simulink/Logic and Bit Operations/Compare To Constant  relop=<  const=32  OutDataTypeStr=boolean
  Compare To Constant1 : simulink/Logic and Bit Operations/Compare To Constant  relop=>  const=27  OutDataTypeStr=boolean
  HDL Counter : hdlsllib/Sources/HDL Counter  CountType=Count limited  CountInit=0  CountStep=1  CountMax=79  CountFromType=Initial value  CountFrom=0  CountResetPort=on  CountLoadPort=off  CountEnbPort=on  CountDirPort=off  CountDataType=Unsigned  CountWordLen=7  CountFracLen=0  CountSampTime=1
  NOT : Logic  Operator=NOT  IconShape=distinctive  AllPortsSameDT=off  OutDataTypeStr=boolean
  y : Outport
  wires:
  NOT/1 -> HDL Counter/1
  enb/1 -> HDL Counter/2, NOT/1
  HDL Counter/1 -> Compare To Constant1/1, Compare To Constant/1
  Compare To Constant/1 -> AND/1
  Compare To Constant1/1 -> AND/2
  AND/1 -> y/1

== system OFDM_Tx_Rx_Loopback/OFDMTx/DataGenerator/LTSfreq ==
  preambVal : Inport
  AND : Logic  IconShape=distinctive  AllPortsSameDT=off  OutDataTypeStr=boolean
  AND1 : Logic  IconShape=distinctive  AllPortsSameDT=off  OutDataTypeStr=boolean
  Compare To Constant : simulink/Logic and Bit Operations/Compare To Constant  relop=>=  const=256  OutDataTypeStr=boolean
  Compare To Constant1 : simulink/Logic and Bit Operations/Compare To Constant  relop=<=  const=319  OutDataTypeStr=boolean
  HDL Counter1 : hdlsllib/Sources/HDL Counter  CountType=Count limited  CountInit=0  CountStep=1  CountMax=319  CountFromType=Initial value  CountFrom=0  CountResetPort=on  CountLoadPort=off  CountEnbPort=on  CountDirPort=off  CountDataType=Unsigned  CountWordLen=9  CountFracLen=0  CountSampTime=1
  HDL Counter4 : hdlsllib/Sources/HDL Counter  CountType=Count limited  CountInit=0  CountStep=1  CountMax=63  CountFromType=Initial value  CountFrom=0  CountResetPort=off  CountLoadPort=off  CountEnbPort=on  CountDirPort=off  CountDataType=Unsigned  CountWordLen=6  CountFracLen=0  CountSampTime=1
  LTSFreq : Lookup_n-D  NumberOfTableDimensions=1  LookupTableObject=''  BreakpointsForDimension1=0:63  BreakpointsForDimension1FirstPoint=10  BreakpointsForDimension2FirstPoint=10  BreakpointsForDimension1Spacing=12  BreakpointsForDimension2Spacing=12  IndexSearchMethod=Evenly spaced points  Table=LTSfreq  TableDataTypeStr=fixdt(1,16,14)  InterpMethod=Flat  DiagnosticForOutOfRangeInput=Error  InternalRulePriority=Speed  OutDataTypeStr=fixdt(1,16,14)  RndMeth=Simplest  InputSameDT=on
  NOT : Logic  Operator=NOT  IconShape=distinctive  AllPortsSameDT=off  OutDataTypeStr=boolean
  ltsFreq : Outport  VectorParamsAs1DForOutWhenUnconnected=off
  ltsVal : Outport  Port=2  VectorParamsAs1DForOutWhenUnconnected=off
  wires:
  HDL Counter4/1 -> LTSFreq/1
  Compare To Constant/1 -> AND/1
  HDL Counter1/1 -> Compare To Constant1/1, Compare To Constant/1
  Compare To Constant1/1 -> AND/2
  NOT/1 -> HDL Counter1/1
  AND/1 -> AND1/1
  preambVal/1 -> NOT/1, AND1/2, HDL Counter1/2
  AND1/1 -> ltsVal/1, HDL Counter4/1
  LTSFreq/1 -> ltsFreq/1

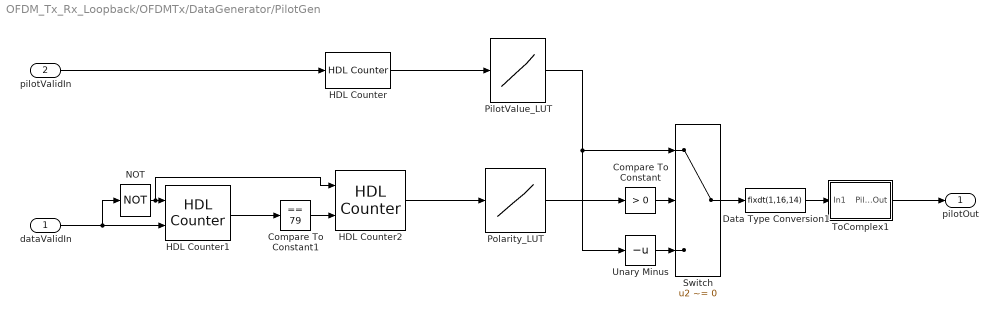
== system OFDM_Tx_Rx_Loopback/OFDMTx/DataGenerator/PilotGen ==
  dataValidIn : Inport
  pilotValidIn : Inport  Port=2
  Compare To Constant : simulink/Logic and Bit Operations/Compare To Constant  relop=>  const=0  OutDataTypeStr=boolean
  Compare To Constant1 : simulink/Logic and Bit Operations/Compare To Constant  relop===  const=79  OutDataTypeStr=boolean
  Data Type Conversion1 : DataTypeConversion  OutDataTypeStr=fixdt(1,16,14)
  HDL Counter : hdlsllib/Sources/HDL Counter  CountType=Count limited  CountInit=0  CountStep=1  CountMax=3  CountFromType=Initial value  CountFrom=0  CountResetPort=off  CountLoadPort=off  CountEnbPort=on  CountDirPort=off  CountDataType=Unsigned  CountWordLen=2  CountFracLen=0  CountSampTime=1
  HDL Counter1 : hdlsllib/Sources/HDL Counter  CountType=Count limited  CountInit=0  CountStep=1  CountMax=79  CountFromType=Initial value  CountFrom=0  CountResetPort=on  CountLoadPort=off  CountEnbPort=on  CountDirPort=off  CountDataType=Unsigned  CountWordLen=8  CountFracLen=0  CountSampTime=1
  HDL Counter2 : hdlsllib/Sources/HDL Counter  CountType=Count limited  CountInit=0  CountStep=1  CountMax=126  CountFromType=Initial value  CountFrom=0  CountResetPort=on  CountLoadPort=off  CountEnbPort=on  CountDirPort=off  CountDataType=Unsigned  CountWordLen=7  CountFracLen=0  CountSampTime=1
  NOT : Logic  Operator=NOT  IconShape=distinctive  AllPortsSameDT=off  OutDataTypeStr=boolean
  PilotValue_LUT : Lookup_n-D  NumberOfTableDimensions=1  LookupTableObject=''  BreakpointsForDimension1=[0:3]  BreakpointsForDimension1FirstPoint=10  BreakpointsForDimension2FirstPoint=10  BreakpointsForDimension1Spacing=12  BreakpointsForDimension2Spacing=12  IndexSearchMethod=Evenly spaced points  Table=[1 1 1 -1]  TableDataTypeStr=fixdt(1,2,0)  InterpMethod=Flat  DiagnosticForOutOfRangeInput=Error  InternalRulePriority=Speed  OutDataTypeStr=fixdt(1,2,0)  RndMeth=Simplest  InputSameDT=on
  Polarity_LUT : Lookup_n-D  NumberOfTableDimensions=1  LookupTableObject=''  BreakpointsForDimension1=[0:126]  BreakpointsForDimension1FirstPoint=10  BreakpointsForDimension2FirstPoint=10  BreakpointsForDimension1Spacing=12  BreakpointsForDimension2Spacing=12  IndexSearchMethod=Evenly spaced points  Table=pilot  TableDataTypeStr=fixdt(1,2,0)  InterpMethod=Flat  DiagnosticForOutOfRangeInput=Error  InternalRulePriority=Speed  OutDataTypeStr=fixdt(1,2,0)  RndMeth=Simplest  InputSameDT=on
  Switch : Switch  Criteria=u2 ~= 0
  ToComplex1 : Subsystem
  Unary Minus : UnaryMinus
  pilotOut : Outport  VectorParamsAs1DForOutWhenUnconnected=off
  wires:
  HDL Counter/1 -> PilotValue_LUT/1
  pilotValidIn/1 -> HDL Counter/1
  Compare To Constant/1 -> Switch/2
  Polarity_LUT/1 -> Compare To Constant/1
  PilotValue_LUT/1 -> Switch/1, Unary Minus/1
  Unary Minus/1 -> Switch/3
  Switch/1 -> Data Type Conversion1/1
  Data Type Conversion1/1 -> ToComplex1/1(In1)
  dataValidIn/1 -> HDL Counter1/2, NOT/1
  HDL Counter1/1 -> Compare To Constant1/1
  NOT/1 -> HDL Counter2/1, HDL Counter1/1
  Compare To Constant1/1 -> HDL Counter2/2
  HDL Counter2/1 -> Polarity_LUT/1
  ToComplex1/1(PilotOut) -> pilotOut/1

== system OFDM_Tx_Rx_Loopback/OFDMTx/DataGenerator/STSFreq ==
  preamVal : Inport
  AND : Logic  IconShape=distinctive  AllPortsSameDT=off  OutDataTypeStr=boolean
  AND1 : Logic  IconShape=distinctive  AllPortsSameDT=off  OutDataTypeStr=boolean
  Compare To Constant : simulink/Logic and Bit Operations/Compare To Constant  relop=>=  const=96  OutDataTypeStr=boolean
  Compare To Constant1 : simulink/Logic and Bit Operations/Compare To Constant  relop=<=  const=159  OutDataTypeStr=boolean
  HDL Counter : hdlsllib/Sources/HDL Counter  CountType=Count limited  CountInit=0  CountStep=1  CountMax=63  CountFromType=Initial value  CountFrom=0  CountResetPort=off  CountLoadPort=off  CountEnbPort=on  CountDirPort=off  CountDataType=Unsigned  CountWordLen=6  CountFracLen=0  CountSampTime=1
  HDL Counter1 : hdlsllib/Sources/HDL Counter  CountType=Count limited  CountInit=0  CountStep=1  CountMax=319  CountFromType=Initial value  CountFrom=0  CountResetPort=on  CountLoadPort=off  CountEnbPort=on  CountDirPort=off  CountDataType=Unsigned  CountWordLen=9  CountFracLen=0  CountSampTime=1
  NOT : Logic  Operator=NOT  IconShape=distinctive  AllPortsSameDT=off  OutDataTypeStr=boolean
  STSFreq : Lookup_n-D  NumberOfTableDimensions=1  LookupTableObject=''  BreakpointsForDimension1=[0:63]  BreakpointsForDimension1FirstPoint=10  BreakpointsForDimension2FirstPoint=10  BreakpointsForDimension1Spacing=12  BreakpointsForDimension2Spacing=12  IndexSearchMethod=Evenly spaced points  Table=STSfreq  TableDataTypeStr=fixdt(1,16,14)  InterpMethod=Flat  DiagnosticForOutOfRangeInput=Error  InternalRulePriority=Speed  OutDataTypeStr=fixdt(1,16,14)  RndMeth=Simplest  InputSameDT=on
  stsFreq : Outport  VectorParamsAs1DForOutWhenUnconnected=off
  stsVal : Outport  Port=2  VectorParamsAs1DForOutWhenUnconnected=off
  wires:
  HDL Counter/1 -> STSFreq/1
  AND/1 -> AND1/1
  HDL Counter1/1 -> Compare To Constant1/1, Compare To Constant/1
  NOT/1 -> HDL Counter1/1
  Compare To Constant/1 -> AND/1
  Compare To Constant1/1 -> AND/2
  preamVal/1 -> NOT/1, AND1/2, HDL Counter1/2
  AND1/1 -> stsVal/1, HDL Counter/1
  STSFreq/1 -> stsFreq/1

== system OFDM_Tx_Rx_Loopback/OFDMTx/DataGenerator/SymbolsGen ==
  modScheme : Inport
  valid : Inport  Port=2
  BPSKmap : Subsystem
  DataGenerator : Subsystem
  DataGenerator1 : Subsystem
  DataGenerator2 : Subsystem  Commented=on
  DataGenerator3 : Subsystem
  Multiport Switch : MultiPortSwitch  DataPortOrder=Zero-based contiguous  zeroidx=on
  QPSKMap : Subsystem
  QPSKMap1 : Subsystem
  symbsOut : Outport  VectorParamsAs1DForOutWhenUnconnected=off
  wires:
  BPSKmap/1(BPSKOut) -> Multiport Switch/2
  modScheme/1 -> Multiport Switch/1
  Multiport Switch/1 -> symbsOut/1
  QPSKMap/1(QPSKOut) -> Multiport Switch/3
  QPSKMap1/1(16QAM) -> Multiport Switch/4
  DataGenerator3/1(bits) -> QPSKMap1/1(ints)
  DataGenerator3/2(validOut) -> QPSKMap1/2(validIn)
  DataGenerator1/1(bits) -> QPSKMap/1(ints)
  DataGenerator1/2(validOut) -> QPSKMap/2(validIn)
  DataGenerator/1(bits) -> BPSKmap/1(bits)
  DataGenerator/2(validOut) -> BPSKmap/2(validIn)
  valid/1 -> DataGenerator3/1(ready), DataGenerator1/1(ready), DataGenerator/1(ready)

== system OFDM_Tx_Rx_Loopback/OFDMTx/IFFT/IFFTValid ==
  preambleValid : Inport
  dataValid : Inport  Port=2
  Switch : Switch  Criteria=u2 ~= 0
  dataIFFTValid : Subsystem
  preambIFFTValid : Subsystem
  ifftValid : Outport  VectorParamsAs1DForOutWhenUnconnected=off
  wires:
  preambleValid/1 -> Switch/2, preambIFFTValid/1(preambValid)
  preambIFFTValid/1(preambIFFTValidOut) -> Switch/1
  dataValid/1 -> dataIFFTValid/1(dataValidIn)
  dataIFFTValid/1(dataIFFTValidOut) -> Switch/3
  Switch/1 -> ifftValid/1

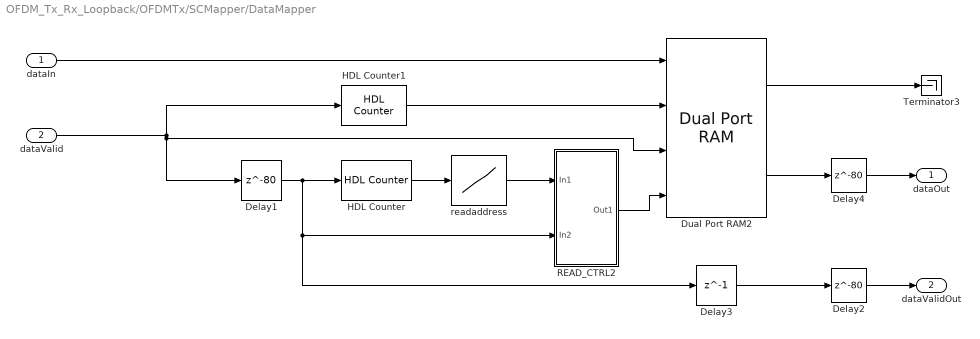
== system OFDM_Tx_Rx_Loopback/OFDMTx/SCMapper/DataMapper ==
  dataIn : Inport
  dataValid : Inport  Port=2
  Delay1 : Delay  DelayLength=80  InitialCondition=0  UseCircularBuffer=on
  Delay2 : Delay  DelayLength=80
  Delay3 : Delay  DelayLength=1  InitialCondition=0  UseCircularBuffer=on
  Delay4 : Delay  DelayLength=80
  Dual Port RAM2 : hdlsllib/HDL RAMs/Dual Port RAM  ram_size=8
      settings: SourceProductBaseCode=SL
  HDL Counter : hdlsllib/Sources/HDL Counter  CountType=Count limited  CountInit=0  CountStep=1  CountMax=159  CountFromType=Initial value  CountFrom=0  CountResetPort=off  CountLoadPort=off  CountEnbPort=on  CountDirPort=off  CountDataType=Unsigned  CountWordLen=8  CountFracLen=0  CountSampTime=1
  HDL Counter1 : hdlsllib/Sources/HDL Counter  CountType=Count limited  CountInit=0  CountStep=1  CountMax=159  CountFromType=Initial value  CountFrom=0  CountResetPort=off  CountLoadPort=off  CountEnbPort=on  CountDirPort=off  CountDataType=Unsigned  CountWordLen=8  CountFracLen=0  CountSampTime=1
  READ_CTRL2 : Subsystem
  Terminator3 : Terminator
  readaddress : Lookup_n-D  NumberOfTableDimensions=1  LookupTableObject=''  BreakpointsForDimension1=[0:159]  BreakpointsForDimension1FirstPoint=10  BreakpointsForDimension2FirstPoint=10  BreakpointsForDimension1Spacing=12  BreakpointsForDimension2Spacing=12  IndexSearchMethod=Evenly spaced points  Table=read_addr_data  TableDataTypeStr=fixdt(0,8,0)  InterpMethod=Flat  DiagnosticForOutOfRangeInput=Error  InternalRulePriority=Speed  OutDataTypeStr=fixdt(0,8,0)  RndMeth=Simplest  InputSameDT=on
  dataOut : Outport  VectorParamsAs1DForOutWhenUnconnected=off
  dataValidOut : Outport  Port=2  VectorParamsAs1DForOutWhenUnconnected=off
  wires:
  READ_CTRL2/1(Out1) -> Dual Port RAM2/4
  Delay3/1 -> Delay2/1
  dataValid/1 -> HDL Counter1/1, Delay1/1, Dual Port RAM2/3
  Dual Port RAM2/2 -> Delay4/1
  Delay1/1 -> READ_CTRL2/2(In2), Delay3/1, HDL Counter/1
  HDL Counter1/1 -> Dual Port RAM2/2
  dataIn/1 -> Dual Port RAM2/1
  HDL Counter/1 -> readaddress/1
  readaddress/1 -> READ_CTRL2/1(In1)
  Dual Port RAM2/1 -> Terminator3/1
  Delay2/1 -> dataValidOut/1
  Delay4/1 -> dataOut/1

== system OFDM_Tx_Rx_Loopback/OFDMTx/SCMapper/PremableMapper ==
  data : Inport
  preambVal : Inport  Port=2
  Delay : Delay  DelayLength=160  InitialCondition=0  UseCircularBuffer=on
  Delay12 : Delay  DelayLength=1  InitialCondition=0  UseCircularBuffer=on
  Dual Port RAM : hdlsllib/HDL RAMs/Dual Port RAM  ram_size=9
      settings: SourceProductBaseCode=SL
  HDL Counter2 : hdlsllib/Sources/HDL Counter  CountType=Count limited  CountInit=0  CountStep=1  CountMax=319  CountFromType=Initial value  CountFrom=0  CountResetPort=off  CountLoadPort=off  CountEnbPort=on  CountDirPort=off  CountDataType=Unsigned  CountWordLen=9  CountFracLen=0  CountSampTime=1
  HDL Counter3 : hdlsllib/Sources/HDL Counter  CountType=Count limited  CountInit=0  CountStep=1  CountMax=319  CountFromType=Initial value  CountFrom=0  CountResetPort=off  CountLoadPort=off  CountEnbPort=on  CountDirPort=off  CountDataType=Unsigned  CountWordLen=9  CountFracLen=0  CountSampTime=1
  READ_CTRL : Subsystem
  Terminator1 : Terminator
  readaddr : Lookup_n-D  NumberOfTableDimensions=1  LookupTableObject=''  BreakpointsForDimension1=0:319  BreakpointsForDimension1FirstPoint=10  BreakpointsForDimension2FirstPoint=10  BreakpointsForDimension1Spacing=12  BreakpointsForDimension2Spacing=12  IndexSearchMethod=Evenly spaced points  Table=read_addr_pream  TableDataTypeStr=fixdt(0,9,0)  InterpMethod=Flat  DiagnosticForOutOfRangeInput=Error  InternalRulePriority=Speed  OutDataTypeStr=fixdt(0,9,0)  RndMeth=Simplest  InputSameDT=on
  preambleShiftOut : Outport  VectorParamsAs1DForOutWhenUnconnected=off
  preambValOut : Outport  Port=2  VectorParamsAs1DForOutWhenUnconnected=off
  wires:
  readaddr/1 -> READ_CTRL/1(In1)
  preambVal/1 -> Delay/1, Dual Port RAM/3, HDL Counter3/1
  READ_CTRL/1(Out1) -> Dual Port RAM/4
  HDL Counter3/1 -> Dual Port RAM/2
  Delay/1 -> READ_CTRL/2(In2), Delay12/1, HDL Counter2/1
  Dual Port RAM/1 -> Terminator1/1
  Delay12/1 -> preambValOut/1
  HDL Counter2/1 -> readaddr/1
  data/1 -> Dual Port RAM/1
  Dual Port RAM/2 -> preambleShiftOut/1
